simulink model "Galvo_sys_v12"  (R2013a)
settings: Solver=ode45  StartTime=0.0  StopTime=30e-3  MaxStep=1e-5  RelTol=1e-3
PreLoadFcn:
  | %Tfin = get_param(gcs,'Tfin');
  | %Kp_cc = evalin('base',paramCtrl.Kp_cc);
  | %CC_EN = 1;
  | %Kp_ccMod = Kp_cc;
PostLoadFcn:
  | %scopes = find_system(gcs, 'BlockType', 'SignalViewerScope');
  | 
  | %for i=1:length(scopes)
  | %  set_param(scopes{i},'open','off');
  | %end
InitFcn:
  | Kp3=evalin('base',paramCtrl.Kp3)
  | %Kp_ccMod = Kp_cc*CC_EN;
  | Tfin=evalin('base','Tfin');
StartFcn:
  | Tfin=evalin('base','Tfin');
model workspace (MATLAB code in the model file):
  | set_param(gcs,'Tfin',num2str(evalin('base', 'Tfin')));
  | Tfin=str2num(get_param(gcs,'Tfin'));
  | CC_EN = 1
  | Kp3=1
values from neighbouring files (symbols this model uses):
  paramCtrl = loadCtrlParam([])    [GalvoModel_v4_sys.m]    (also in Galvo_process_analyze.m = loadCtrlParam(4))
libraries: simulink x2
settings Model: CC_EN=1  Tfin=0.01  TunableVars=Kp3  TunableVarsStorageClass=Auto  BufferReuse=off  Creator=mainster  LastModifiedBy=mainster
settings DataIOCC: LimitDataPoints=off  SaveOutput=off  SignalLogging=off  DSMLogging=off  SaveTime=off
settings OptimizationCC: BlockReduction=off  InlineParams=on  InlineInvariantSignals=on  OptimizeBlockIOStorage=off  BufferReuse=off  ExpressionFolding=off  LocalBlockOutputs=off
settings DebuggingCC: InitInArrayFormatMsg=none

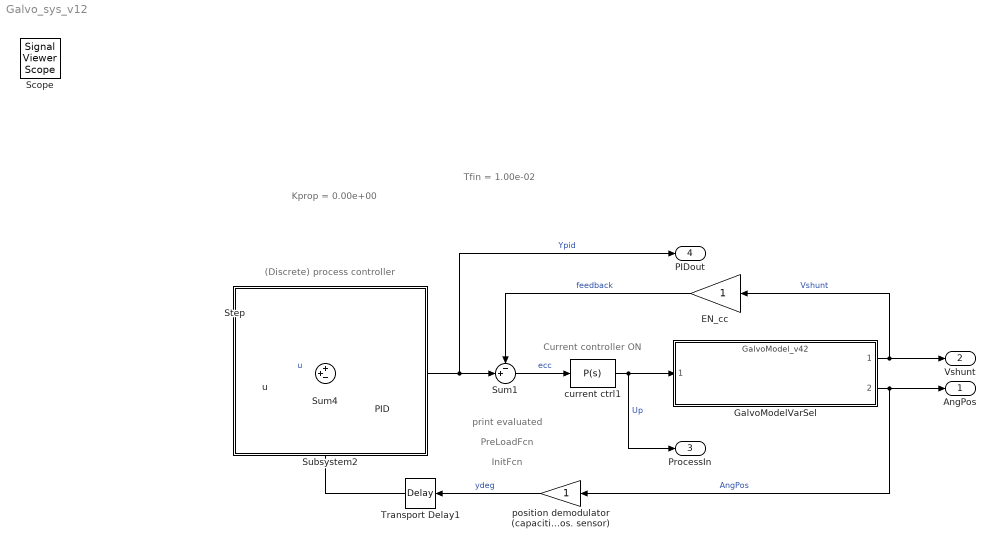
== system Galvo_sys_v12 ==
  note: Tfin = 1.00e-02
  note: Kprop = 0.00e+00
  note: (Discrete) process controller
  note: Current controller ON
  note: print evaluated
  note: PreLoadFcn
  note: InitFcn
  u : Inport
  EN_cc : Gain
  GalvoModelVarSel : ModelReference  ModelNameDialog=GalvoModel_v42.slx  SimulationMode=Normal  OverrideUsingVariant=Galvo_v42  ModelReferenceVersion=1.13  CopyOfModelName=GalvoModel_v42.slx  DefaultDataLogging=on
      mask init:
      | % 
      | % evalin('base', ['param=loadGalvoParam(' strrep(modVers(2:end-1),'.','') ');'])
      | % 
      | % switch modVers(1:2)
      | %     case 'v4'
      | %                 JR=evalin('base','param.JR');
      | %                 KMT=evalin('base','param.KMT');
      | %                 Rc=evalin('base','param.Rc');
      | %                 Lc=evalin('base','param.Lc');
      | %                 KFR=evalin('base','param.KFR');
      | %                 KTB=evalin('base','param.KTB');
      | %                 KBM=evalin('base','param.KBM');
      | %                 Rsh=evalin('base','param.Rsh');
      | %     case 'v3'
      | % 
      | %                 RIN=evalin('base','param.RIN');
      | %                 TRC=evalin('base','param.TRC');
      | %                 CR=evalin('base','param.CR');
      | %                 CL=evalin('base','param.CL');
      | %                 FR=evalin('base','param.FR');
      | %                 KTR=evalin('base','param.KTR');
      | %                 BEM=evalin('base','param.BEM');
      | %                 SHR=evalin('base','param.SHR');
      | %     otherwise
      | % 
      | % end
      | % 
      | % set_param(gcb, 'OverrideUsingVariant',sprintf('Galvo_%s',strrep(modVers,'.','')))
      | %
      settings: AttributesFormatString=%<ActiveVariant>\n%<Name>\n%<Name>\n%<NamePlacement>
      mask Display:
      | str=sprintf('%s',get(gcbh,'ModelName'));
      | port_label('input', 1, 'VCoil','texmode','on')
      | color('blue');
      | port_label('output', 1, 'VShunt','texmode','on')
      | color('black');
      | port_label('output', 2, 'AngPos')
      | %text(.05,.98,['{\fontsize{12}\it\bf' strrep(str,'_',' ') '}'],'horizontalAlignment','left','verticalAlignment','top','texmode','on')
      | text(.015,.98,['{\fontsize{12}\it\bf' strrep(str,'_','\_') '}'],'horizontalAlignment','left','verticalAlignment','top','texmode','on')
  PID : simulink/Continuous/PID Controller  Controller=PID  TimeDomain=Continuous-time  SampleTime=1  IntegratorMethod=Forward Euler  FilterMethod=Forward Euler  Form=Ideal  P=1.14533423709275  I=9.52023676976267  D=0.0126974512595782  N=3428.84832659657  InitialConditionSource=internal  InitialConditionForIntegrator=0  InitialConditionForFilter=0  ExternalReset=none  IgnoreLimit=on  LimitOutput=on  UpperSaturationLimit=2.5  LowerSaturationLimit=-2.5  LinearizeAsGain=on  AntiWindupMode=back-calculation  Kb=6  TrackingMode=off  Kt=0  PParamMin=[]  PParamMax=[]  IParamMin=[]  IParamMax=[]  DParamMin=[]  DParamMax=[]  NParamMin=[]  NParamMax=[]  KbParamMin=[]  KbParamMax=[]  KtParamMin=[]  KtParamMax=[]  POutMin=[]  POutMax=[]  IOutMin=[]  IOutMax=[]  DOutMin=[]  DOutMax=[]  NOutMin=[]  NOutMax=[]  KbOutMin=[]  KbOutMax=[]  KtOutMin=[]  KtOutMax=[]  IntegratorOutMin=[]  IntegratorOutMax=[]  FilterOutMin=[]  FilterOutMax=[]  SumOutMin=[]  SumOutMax=[]  SumI1OutMin=[]  SumI1OutMax=[]  SumI2OutMin=[]  SumI2OutMax=[]  SumI3OutMin=[]  SumI3OutMax=[]  SumDOutMin=[]  SumDOutMax=[]  SaturationOutMin=[]  SaturationOutMax=[]  IntegratorContinuousStateAttributes=''  IntegratorStateMustResolveToSignalObject=off  IntegratorRTWStateStorageClass=Auto  FilterContinuousStateAttributes=''  FilterStateMustResolveToSignalObject=off  FilterRTWStateStorageClass=Auto
  Step : Step  Time=1e-3  SampleTime=0  ZeroCross=off
      settings: AttributesFormatString=Ampl.: %<After>
  Subsystem2 : Subsystem  mask{d=0}
      mask Display: disp('')
  Sum1 : Sum  Inputs=-+|
  Sum4 : Sum  Inputs=++-
  Transport Delay1 : TransportDelay  DelayTime=1e-6
  current ctrl1 : simulink/Continuous/PID Controller  Controller=P  TimeDomain=Continuous-time  SampleTime=1  IntegratorMethod=Forward Euler  FilterMethod=Forward Euler  Form=Ideal  P=Kp3  I=0.7525  D=0.156  N=100  InitialConditionSource=internal  InitialConditionForIntegrator=0  InitialConditionForFilter=0  ExternalReset=none  ZeroCross=off  LimitOutput=on  UpperSaturationLimit=25  LowerSaturationLimit=-25  LinearizeAsGain=on  AntiWindupMode=none  Kb=1  TrackingMode=off  Kt=1  PParamMin=[]  PParamMax=[]  IParamMin=[]  IParamMax=[]  DParamMin=[]  DParamMax=[]  NParamMin=[]  NParamMax=[]  KbParamMin=[]  KbParamMax=[]  KtParamMin=[]  KtParamMax=[]  POutMin=[]  POutMax=[]  IOutMin=[]  IOutMax=[]  DOutMin=[]  DOutMax=[]  NOutMin=[]  NOutMax=[]  KbOutMin=[]  KbOutMax=[]  KtOutMin=[]  KtOutMax=[]  IntegratorOutMin=[]  IntegratorOutMax=[]  FilterOutMin=[]  FilterOutMax=[]  SumOutMin=[]  SumOutMax=[]  SumI1OutMin=[]  SumI1OutMax=[]  SumI2OutMin=[]  SumI2OutMax=[]  SumI3OutMin=[]  SumI3OutMax=[]  SumDOutMin=[]  SumDOutMax=[]  SaturationOutMin=[]  SaturationOutMax=[]  IntegratorContinuousStateAttributes=''  IntegratorStateMustResolveToSignalObject=off  IntegratorRTWStateStorageClass=Auto  FilterContinuousStateAttributes=''  FilterStateMustResolveToSignalObject=off  FilterRTWStateStorageClass=Auto
  position demodulator (capacitive angular pos. sensor) : Gain
  AngPos : Outport
  Vshunt : Outport  Port=2
  ProcessIn : Outport  Port=3
  PIDout : Outport  Port=4
  Scope : SignalViewerScope  IOType=viewer  NumInputPorts=4  LegendLocations=|  RefreshTime=0.035000
      | 0.83411     0.93642     0.12035    0.021645
      | 0.86602     0.70049    0.088431    0.021645
      | 0.85007     0.44656     0.10439    0.038555
      | 0.83411     0.22754     0.12035    0.021645
      settings: ShowLegends=on  TimeRange=0.03  YMin=-0.2~-2~-2~-0.1  YMax=1~3~3~0.15  MaxDataPoints=75000
  wires:
  Sum4/1 -> PID/1
  Step/1 -> Sum4/1
  u/1 -> Sum4/2  "u"
  position demodulator (capacitive angular pos. sensor)/1 -> Transport Delay1/1  "ydeg"
  Sum1/1 -> current ctrl1/1  "ecc"
  GalvoModelVarSel/1 -> Vshunt/1, EN_cc/1  "Vshunt"
  current ctrl1/1 -> ProcessIn/1, GalvoModelVarSel/1  "Up"
  PID/1 -> PIDout/1, Sum1/2  "Ypid"
  GalvoModelVarSel/2 -> AngPos/1, position demodulator (capacitive angular pos. sensor)/1  "AngPos"
  EN_cc/1 -> Sum1/1  "feedback"
  Transport Delay1/1 -> Sum4/3

== system Galvo_sys_v12/Subsystem2 ==
